simulink model "Simple_3_Model"  (R2022b)
settings: Solver=FixedStepAuto  StartTime=0.0  StopTime=1000  FixedStep=.05  RelTol=1e-3
undefined symbols (not defined in the file or in its folder): importedData
libraries: matrix_library x9
(part 1 of 2)
settings Model: SimulationMode=accelerator  Creator=hollis  LastModifiedBy=hollis
settings ModelReferenceCC: EnableRefExpFcnMdlSchedulingChecks=on

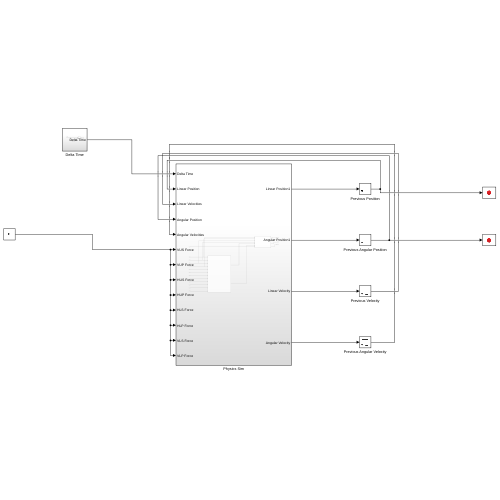
[thumbnail: Simulink's stored preview of the top-level diagram]
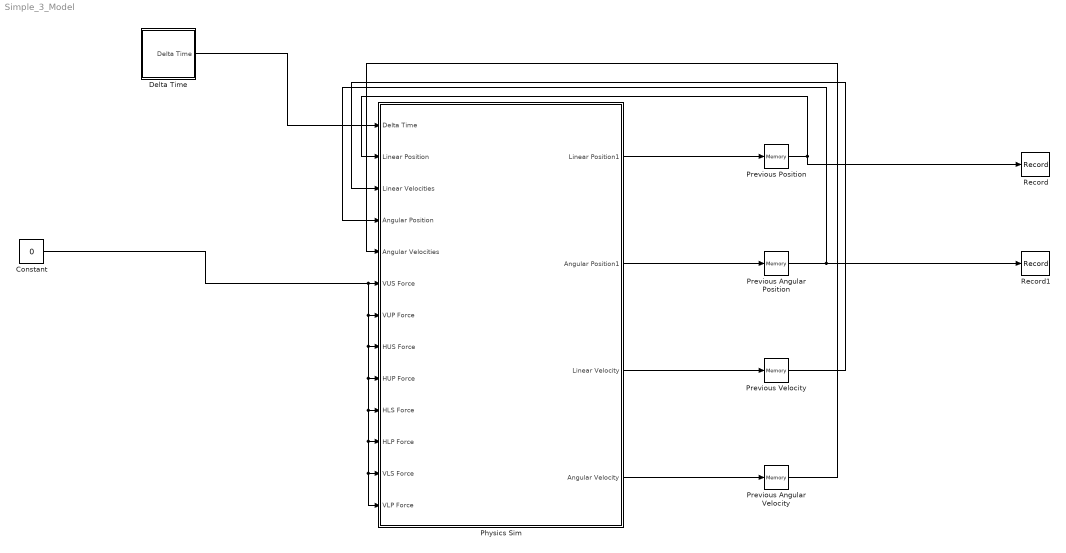
== system Simple_3_Model ==
  Constant : Constant  Value=0
  Delta Time : Subsystem
  Physics Sim : Subsystem
  Previous Angular Position : Memory
  Previous Angular Velocity : Memory
  Previous Position : Memory  InitialCondition=[0,0,-1]
  Previous Velocity : Memory
  Record : Record  FileSettingsInternal="{\"entries\":[{\"content\":{\"excelSettings\":{\"content\":{},\"type\":\"Streamout.ExcelSettings\"}},\"type\":\"Streamout.FileSettingStorage\",\"uuid\":\"11bcd66e-7632-4a96-a488-3543fce7ee1d\"}],\"packageUris\":[\"http://schema.mathworks.com/mf0/streamout_blocks/R2020a\"],\"version\":\"1.0\"}"  SignalsInternal="{\"entries\":[{\"content\":{\"signals\":[{\"content\":{\"blockPath\":[\"Simple_3_Model/Record\"],\"channel\":[],\"dimensions\":[1,3],\"domain\":\"Simple_3_Model/Record\",\"hasChildren\":true,\"lineColor\":\"#fe330a\",\"plots\":[],\"port\":1,\"sid\":[\"\"],\"signalID\":926,\"signalName\":\"Previous Position\"},\"type\":\"RecordBlkView.Signal\",\"uuid\":\"373110d8-16e4-4d5b-b50e-cea3cb7c1b6c\"},{\"content\":{\"blockPath\":[\"Simple_3_Model/Record\"],\"channel\":[1,1],\"dimensions\":[1,3],\"domain\":\"Simple_3_Model/Record\",\"lineColor\":\"#d95319\",\"parentID\":926,\"plots\":[1],\"port\":1,\"sid\":[\"\"],\"signalID\":927,\"signalName\":\"Previous Position\"},\"type\":\"RecordBlkView.Signal\",\"uuid\":\"bcdab5c0-74a8-478b-9c24-691629be9185\"},{\"content\":{\"blockPath\":[\"Simple_3_Model/Record\"],\"channel\":[1,2],\"dimensions\":[1,3],\"domain\":\"Simple_3_Model/Record\",\"lineColor\":\"#22b573\",\"parentID\":926,\"plots\":[1],\"port\":1,\"sid\":[\"\"],\"signalID\":965,\"signalName\":\"Previous Position\"},\"type\":\"RecordBlkView.Signal\",\"uuid\":\"4fc746e4-520d-4283-b26c-b6a945fd0e94\"},{\"content\":{\"blockPath\":[\"Simple_3_Model/Record\"],\"channel\":[1,3],\"dimensions\":[1,3],\"domain\":\"Simple_3_Model/Record\",\"lineColor\":\"#0072bd\",\"parentID\":926,\"plots\":[1],\"port\":1,\"sid\":[\"\"],\"signalID\":966,\"signalName\":\"Previous Position\"},\"type\":\"RecordBlkView.Signal\",\"uuid\":\"20b07a7b-441e-4fa1-b232-437ed8d86cd2\"}]},\"type\":\"RecordBlkView.InputSignals\",\"uuid\":\"0cc5a42f-1473-481d-9a59-2aee6edbe01c\"}],\"packageUris\":[\"http://schema.mathworks.com/mf0/streamout_blocks/R2020a\"],\"version\":\"1.0\"}"  VisualizationBindings="{\"sparklinesplugin\":{\"info\":[{\"bindingParametersList\":[],\"subplotID\":1}]}}"
  Record1 : Record  FileSettingsInternal="{\"entries\":[{\"content\":{\"excelSettings\":{\"content\":{},\"type\":\"Streamout.ExcelSettings\"}},\"type\":\"Streamout.FileSettingStorage\",\"uuid\":\"971a0b71-2232-4346-b6ce-2804bd4b2a6a\"}],\"packageUris\":[\"http://schema.mathworks.com/mf0/streamout_blocks/R2020a\"],\"version\":\"1.0\"}"  SignalsInternal="{\"entries\":[{\"content\":{\"signals\":[{\"content\":{\"blockPath\":[\"Simple_3_Model/Record1\"],\"channel\":[],\"dimensions\":[1,3],\"domain\":\"Simple_3_Model/Record1\",\"hasChildren\":true,\"lineColor\":\"#0072bd\",\"plots\":[],\"port\":1,\"sid\":[\"\"],\"signalID\":931,\"signalName\":\"Previous Angular Position\"},\"type\":\"RecordBlkView.Signal\",\"uuid\":\"942ad879-51dd-44a6-9b93-fffe35835e0f\"},{\"content\":{\"blockPath\":[\"Simple_3_Model/Record1\"],\"channel\":[1,1],\"dimensions\":[1,3],\"domain\":\"Simple_3_Model/Record1\",\"lineColor\":\"#0072bd\",\"parentID\":931,\"plots\":[1],\"port\":1,\"sid\":[\"\"],\"signalID\":932,\"signalName\":\"Previous Angular Position\"},\"type\":\"RecordBlkView.Signal\",\"uuid\":\"0f7508f4-6f39-4d77-9981-5362550e1fb4\"},{\"content\":{\"blockPath\":[\"Simple_3_Model/Record1\"],\"channel\":[1,2],\"dimensions\":[1,3],\"domain\":\"Simple_3_Model/Record1\",\"lineColor\":\"#0072bd\",\"parentID\":931,\"plots\":[1],\"port\":1,\"sid\":[\"\"],\"signalID\":967,\"signalName\":\"Previous Angular Position\"},\"type\":\"RecordBlkView.Signal\",\"uuid\":\"f8e5f5da-daa1-4c33-b5ed-8b7ecbecee5a\"},{\"content\":{\"blockPath\":[\"Simple_3_Model/Record1\"],\"channel\":[1,3],\"dimensions\":[1,3],\"domain\":\"Simple_3_Model/Record1\",\"lineColor\":\"#d95319\",\"parentID\":931,\"plots\":[1],\"port\":1,\"sid\":[\"\"],\"signalID\":968,\"signalName\":\"Previous Angular Position\"},\"type\":\"RecordBlkView.Signal\",\"uuid\":\"b5832108-d461-432d-a375-5bfff83e6820\"}]},\"type\":\"RecordBlkView.InputSignals\",\"uuid\":\"14037c08-81e6-44a9-86f7-5d7daad76c4f\"}],\"packageUris\":[\"http://schema.mathworks.com/mf0/streamout_blocks/R2020a\"],\"version\":\"1.0\"}"  VisualizationBindings="{\"sparklinesplugin\":{\"info\":[{\"bindingParametersList\":[],\"subplotID\":1}]}}"
  wires:
  Physics Sim/1(Linear Position1) -> Previous Position/1
  Physics Sim/2(Angular Position1) -> Previous Angular Position/1
  Physics Sim/3(Linear Velocity) -> Previous Velocity/1
  Physics Sim/4(Angular Velocity) -> Previous Angular Velocity/1
  Delta Time/1(Delta Time) -> Physics Sim/1(Delta Time)
  Previous Position/1 -> Record/1, Physics Sim/2(Linear Position)
  Previous Angular Position/1 -> Record1/1, Physics Sim/4(Angular Position)
  Previous Velocity/1 -> Physics Sim/3(Linear Velocities)
  Previous Angular Velocity/1 -> Physics Sim/5(Angular Velocities)
  Constant/1 -> Physics Sim/13(VLP Force), Physics Sim/12(VLS Force), Physics Sim/11(HLP Force), Physics Sim/10(HLS Force), Physics Sim/9(HUP Force), Physics Sim/8(HUS Force), Physics Sim/7(VUP Force), Physics Sim/6(VUS Force)

== system Simple_3_Model/Delta Time ==
  Absolute Time : Clock
  Previous Absolute : Memory
  Subtract : Sum  Inputs=+-
  Delta Time : Outport
  wires:
  Previous Absolute/1 -> Subtract/2
  Absolute Time/1 -> Subtract/1, Previous Absolute/1
  Subtract/1 -> Delta Time/1

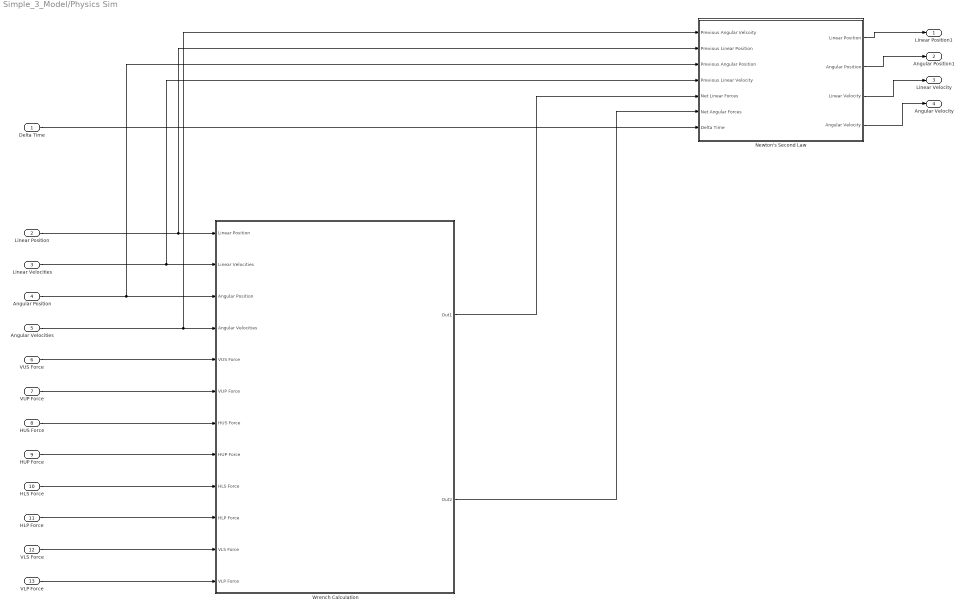
== system Simple_3_Model/Physics Sim ==
  Delta Time : Inport
  Linear Position : Inport  Port=2
  Linear Velocities : Inport  Port=3
  Angular Position : Inport  Port=4
  Angular Velocities : Inport  Port=5
  VUS Force : Inport  Port=6
  VUP Force : Inport  Port=7
  HUS Force : Inport  Port=8
  HUP Force : Inport  Port=9
  HLS Force : Inport  Port=10
  HLP Force : Inport  Port=11
  VLS Force : Inport  Port=12
  VLP Force : Inport  Port=13
  Newton's Second Law : Subsystem
  Wrench Calculation : Subsystem
  Linear Position1 : Outport
  Angular Position1 : Outport  Port=2
  Linear Velocity : Outport  Port=3
  Angular Velocity : Outport  Port=4
  wires:
  Delta Time/1 -> Newton's Second Law/7(Delta Time)
  VLP Force/1 -> Wrench Calculation/12(VLP Force)
  VUP Force/1 -> Wrench Calculation/6(VUP Force)
  Newton's Second Law/3(Linear Velocity) -> Linear Velocity/1
  VUS Force/1 -> Wrench Calculation/5(VUS Force)
  Newton's Second Law/1(Linear Position) -> Linear Position1/1
  Newton's Second Law/4(Angular Velocity) -> Angular Velocity/1
  HLS Force/1 -> Wrench Calculation/9(HLS Force)
  Angular Position/1 -> Newton's Second Law/3(Previous Angular Position), Wrench Calculation/3(Angular Position)
  Newton's Second Law/2(Angular Position) -> Angular Position1/1
  VLS Force/1 -> Wrench Calculation/11(VLS Force)
  HLP Force/1 -> Wrench Calculation/10(HLP Force)
  HUP Force/1 -> Wrench Calculation/8(HUP Force)
  Angular Velocities/1 -> Newton's Second Law/1(Previous Angular Velcoity), Wrench Calculation/4(Angular Velocities)
  Linear Velocities/1 -> Newton's Second Law/4(Previous Linear Velocity), Wrench Calculation/2(Linear Velocities)
  Wrench Calculation/1(Out1) -> Newton's Second Law/5(Net Linear Forces)
  Linear Position/1 -> Newton's Second Law/2(Previous Linear Position), Wrench Calculation/1(Linear Position)
  HUS Force/1 -> Wrench Calculation/7(HUS Force)
  Wrench Calculation/2(Out2) -> Newton's Second Law/6(Net Angular Forces)

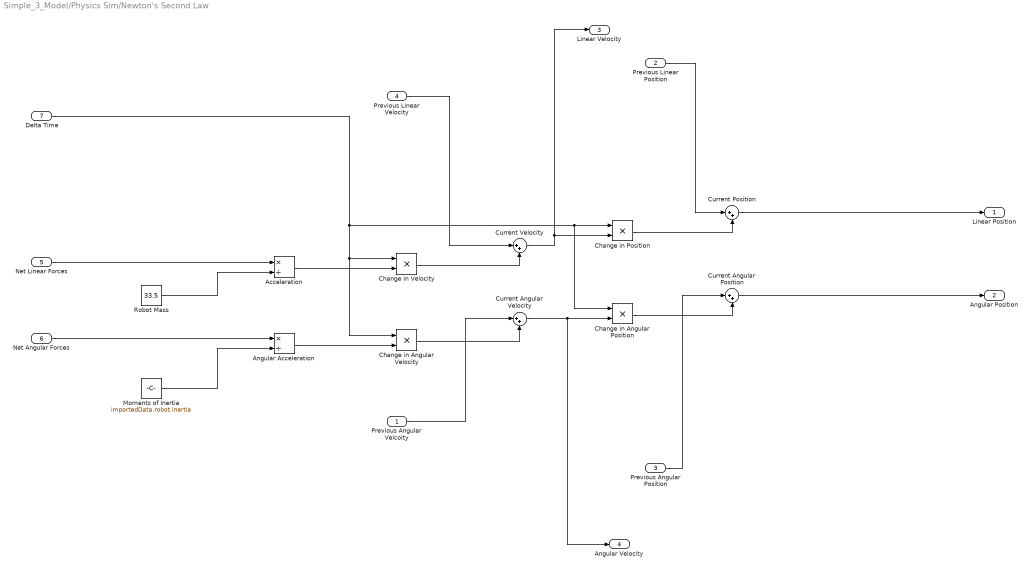
== system Simple_3_Model/Physics Sim/Newton's Second Law ==
  Previous Angular Velcoity : Inport
  Previous Linear Position : Inport  Port=2
  Previous Angular Position : Inport  Port=3
  Previous Linear Velocity : Inport  Port=4
  Net Linear Forces : Inport  Port=5
  Net Angular Forces : Inport  Port=6
  Delta Time : Inport  Port=7
  Acceleration : Product  Inputs=*/
  Angular Acceleration : Product  Inputs=*/
  Change in Angular Position : Product
  Change in Angular Velocity : Product
  Change in Position : Product
  Change in Velocity : Product
  Current Angular Position : Sum  Inputs=|++
  Current Angular Velocity : Sum  Inputs=|++
  Current Position : Sum  Inputs=|++
  Current Velocity : Sum  Inputs=|++
  Moments of Inertia : Constant  Value=importedData.robot.inertia  VectorParams1D=off
  Robot Mass : Constant  Value=33.5
  Linear Position : Outport
  Angular Position : Outport  Port=2
  Linear Velocity : Outport  Port=3
  Angular Velocity : Outport  Port=4
  wires:
  Current Angular Position/1 -> Angular Position/1
  Acceleration/1 -> Change in Velocity/2
  Angular Acceleration/1 -> Change in Angular Velocity/2
  Change in Position/1 -> Current Position/2
  Moments of Inertia/1 -> Angular Acceleration/2
  Current Velocity/1 -> Linear Velocity/1, Change in Position/2
  Current Position/1 -> Linear Position/1
  Previous Linear Velocity/1 -> Current Velocity/1
  Change in Angular Velocity/1 -> Current Angular Velocity/2
  Net Linear Forces/1 -> Acceleration/1
  Net Angular Forces/1 -> Angular Acceleration/1
  Current Angular Velocity/1 -> Angular Velocity/1, Change in Angular Position/2
  Change in Angular Position/1 -> Current Angular Position/2
  Previous Angular Velcoity/1 -> Current Angular Velocity/1
  Delta Time/1 -> Change in Angular Velocity/1, Change in Velocity/1, Change in Angular Position/1, Change in Position/1
  Previous Linear Position/1 -> Current Position/1
  Robot Mass/1 -> Acceleration/2
  Previous Angular Position/1 -> Current Angular Position/1
  Change in Velocity/1 -> Current Velocity/2

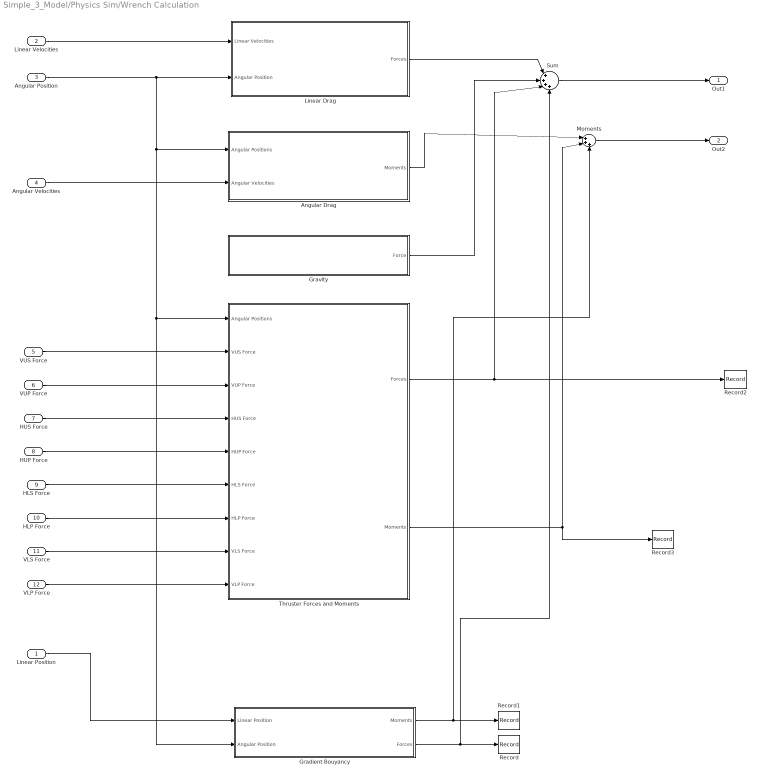
== system Simple_3_Model/Physics Sim/Wrench Calculation ==
  Linear Position : Inport
  Linear Velocities : Inport  Port=2
  Angular Position : Inport  Port=3
  Angular Velocities : Inport  Port=4
  VUS Force : Inport  Port=5
  VUP Force : Inport  Port=6
  HUS Force : Inport  Port=7
  HUP Force : Inport  Port=8
  HLS Force : Inport  Port=9
  HLP Force : Inport  Port=10
  VLS Force : Inport  Port=11
  VLP Force : Inport  Port=12
  Angular Drag : Subsystem
  Gradient Bouyancy : Subsystem
  Gravity : Subsystem
  Linear Drag : Subsystem
  Moments : Sum  Inputs=|+++
  Record : Record  FileSettingsInternal="{\"entries\":[{\"content\":{\"excelSettings\":{\"content\":{},\"type\":\"Streamout.ExcelSettings\"}},\"type\":\"Streamout.FileSettingStorage\",\"uuid\":\"14ae8275-bff0-4191-85a7-8bdbe692570f\"}],\"packageUris\":[\"http://schema.mathworks.com/mf0/streamout_blocks/R2020a\"],\"version\":\"1.0\"}"  SignalsInternal="{\"entries\":[{\"content\":{\"signals\":[{\"content\":{\"blockPath\":[\"Simple_3_Model/Physics Sim/Wrench Calculation/Record\"],\"channel\":[],\"dimensions\":[1,3],\"domain\":\"Simple_3_Model/Physics Sim/Wrench Calculation/Record\",\"hasChildren\":true,\"lineColor\":\"#edb120\",\"plots\":[],\"port\":1,\"sid\":[\"\"],\"signalID\":936,\"signalName\":\"Gradient Bouyancy:2\"},\"type\":\"RecordBlkView.Signal\",\"uuid\":\"7bfce770-828e-487e-b922-719935c79236\"},{\"content\":{\"blockPath\":[\"Simple_3_Model/Physics Sim/Wrench Calculation/Record\"],\"channel\":[1,1],\"dimensions\":[1,3],\"domain\":\"Simple_3_Model/Physics Sim/Wrench Calculation/Record\",\"lineColor\":\"#ff6929\",\"parentID\":936,\"plots\":[1],\"port\":1,\"sid\":[\"\"],\"signalID\":937,\"signalName\":\"Gradient Bouyancy:2\"},\"type\":\"RecordBlkView.Signal\",\"uuid\":\"0b18444a-b670-4689-ba02-5d1e4877daca\"},{\"content\":{\"blockPath\":[\"Simple_3_Model/Physics Sim/Wrench Calculation/Record\"],\"channel\":[1,2],\"dimensions\":[1,3],\"domain\":\"Simple_3_Model/Physics Sim/Wrench Calculation/Record\",\"lineColor\":\"#4dbeee\",\"parentID\":936,\"plots\":[1],\"port\":1,\"sid\":[\"\"],\"signalID\":969,\"signalName\":\"Gradient Bouyancy:2\"},\"type\":\"RecordBlkView.Signal\",\"uuid\":\"a577dcb4-3a6d-43f4-9b39-8c81b2194628\"},{\"content\":{\"blockPath\":[\"Simple_3_Model/Physics Sim/Wrench Calculation/Record\"],\"channel\":[1,3],\"dimensions\":[1,3],\"domain\":\"Simple_3_Model/Physics Sim/Wrench Calculation/Record\",\"lineColor\":\"#a2142f\",\"parentID\":936,\"plots\":[1],\"port\":1,\"sid\":[\"\"],\"signalID\":970,\"signalName\":\"Gradient Bouyancy:2\"},\"type\":\"RecordBlkView.Signal\",\"uuid\":\"bcba812b-f663-473e-a7f6-fe747fcb18b0\"}]},\"type\":\"RecordBlkView.InputSignals\",\"uuid\":\"80eec240-2a13-4c7e-96b9-5123065623d5\"}],\"packageUris\":[\"http://schema.mathworks.com/mf0/streamout_blocks/R2020a\"],\"version\":\"1.0\"}"  VisualizationBindings="{\"sparklinesplugin\":{\"info\":[{\"bindingParametersList\":[],\"subplotID\":1}]}}"
  Record1 : Record  FileSettingsInternal="{\"entries\":[{\"content\":{\"excelSettings\":{\"content\":{},\"type\":\"Streamout.ExcelSettings\"}},\"type\":\"Streamout.FileSettingStorage\",\"uuid\":\"c8ebd48f-3dda-4790-90f8-fdd6d3865a6d\"}],\"packageUris\":[\"http://schema.mathworks.com/mf0/streamout_blocks/R2020a\"],\"version\":\"1.0\"}"  SignalsInternal="{\"entries\":[{\"content\":{\"signals\":[{\"content\":{\"blockPath\":[\"Simple_3_Model/Physics Sim/Wrench Calculation/Record1\"],\"channel\":[],\"dimensions\":[1,3],\"domain\":\"Simple_3_Model/Physics Sim/Wrench Calculation/Record1\",\"hasChildren\":true,\"lineColor\":\"#77ac30\",\"plots\":[],\"port\":1,\"sid\":[\"\"],\"signalID\":941,\"signalName\":\"Gradient Bouyancy:1\"},\"type\":\"RecordBlkView.Signal\",\"uuid\":\"01770711-47fc-4378-9b06-d566efdae185\"},{\"content\":{\"blockPath\":[\"Simple_3_Model/Physics Sim/Wrench Calculation/Record1\"],\"channel\":[1,1],\"dimensions\":[1,3],\"domain\":\"Simple_3_Model/Physics Sim/Wrench Calculation/Record1\",\"lineColor\":\"#64d413\",\"parentID\":941,\"plots\":[1],\"port\":1,\"sid\":[\"\"],\"signalID\":942,\"signalName\":\"Gradient Bouyancy:1\"},\"type\":\"RecordBlkView.Signal\",\"uuid\":\"9acf9cb1-4fa8-4bf8-90f0-6f697aa656da\"},{\"content\":{\"blockPath\":[\"Simple_3_Model/Physics Sim/Wrench Calculation/Record1\"],\"channel\":[1,2],\"dimensions\":[1,3],\"domain\":\"Simple_3_Model/Physics Sim/Wrench Calculation/Record1\",\"lineColor\":\"#139fff\",\"parentID\":941,\"plots\":[1],\"port\":1,\"sid\":[\"\"],\"signalID\":971,\"signalName\":\"Gradient Bouyancy:1\"},\"type\":\"RecordBlkView.Signal\",\"uuid\":\"442f376c-a923-410e-a81f-817bbf379f20\"},{\"content\":{\"blockPath\":[\"Simple_3_Model/Physics Sim/Wrench Calculation/Record1\"],\"channel\":[1,3],\"dimensions\":[1,3],\"domain\":\"Simple_3_Model/Physics Sim/Wrench Calculation/Record1\",\"lineColor\":\"#ff6929\",\"parentID\":941,\"plots\":[1],\"port\":1,\"sid\":[\"\"],\"signalID\":972,\"signalName\":\"Gradient Bouyancy:1\"},\"type\":\"RecordBlkView.Signal\",\"uuid\":\"d23a1b4a-4761-4174-b835-0283a7d905c5\"}]},\"type\":\"RecordBlkView.InputSignals\",\"uuid\":\"540da4e7-907c-4693-a7c6-038eda139879\"}],\"packageUris\":[\"http://schema.mathworks.com/mf0/streamout_blocks/R2020a\"],\"version\":\"1.0\"}"  VisualizationBindings="{\"sparklinesplugin\":{\"info\":[{\"bindingParametersList\":[],\"subplotID\":1}]}}"
  Record2 : Record  FileSettingsInternal="{\"entries\":[{\"content\":{\"excelSettings\":{\"content\":{},\"type\":\"Streamout.ExcelSettings\"}},\"type\":\"Streamout.FileSettingStorage\",\"uuid\":\"6320329a-b3d7-4a3d-9256-9fc55a292c12\"}],\"packageUris\":[\"http://schema.mathworks.com/mf0/streamout_blocks/R2020a\"],\"version\":\"1.0\"}"  SignalsInternal="{\"entries\":[{\"content\":{\"signals\":[{\"content\":{\"blockPath\":[\"Simple_3_Model/Physics Sim/Wrench Calculation/Record2\"],\"channel\":[],\"dimensions\":[1,3],\"domain\":\"Simple_3_Model/Physics Sim/Wrench Calculation/Record2\",\"hasChildren\":true,\"lineColor\":\"#a2142f\",\"plots\":[],\"port\":1,\"sid\":[\"\"],\"signalID\":946,\"signalName\":\"Thruster Forces and Moments:1\"},\"type\":\"RecordBlkView.Signal\",\"uuid\":\"e0bec64a-e0fc-4c30-ba04-1f75709ad5d1\"},{\"content\":{\"blockPath\":[\"Simple_3_Model/Physics Sim/Wrench Calculation/Record2\"],\"channel\":[1,1],\"dimensions\":[1,3],\"domain\":\"Simple_3_Model/Physics Sim/Wrench Calculation/Record2\",\"lineColor\":\"#0072bd\",\"parentID\":946,\"plots\":[1],\"port\":1,\"sid\":[\"\"],\"signalID\":947,\"signalName\":\"Thruster Forces and Moments:1\"},\"type\":\"RecordBlkView.Signal\",\"uuid\":\"92f7a7a3-98ca-4f61-a9f6-ac5a2e273ed5\"},{\"content\":{\"blockPath\":[\"Simple_3_Model/Physics Sim/Wrench Calculation/Record2\"],\"channel\":[1,2],\"dimensions\":[1,3],\"domain\":\"Simple_3_Model/Physics Sim/Wrench Calculation/Record2\",\"lineColor\":\"#ff6929\",\"parentID\":946,\"plots\":[1],\"port\":1,\"sid\":[\"\"],\"signalID\":973,\"signalName\":\"Thruster Forces and Moments:1\"},\"type\":\"RecordBlkView.Signal\",\"uuid\":\"18811a90-2073-45f0-bfd8-044204d09150\"},{\"content\":{\"blockPath\":[\"Simple_3_Model/Physics Sim/Wrench Calculation/Record2\"],\"channel\":[1,3],\"dimensions\":[1,3],\"domain\":\"Simple_3_Model/Physics Sim/Wrench Calculation/Record2\",\"lineColor\":\"#b746ff\",\"parentID\":946,\"plots\":[1],\"port\":1,\"sid\":[\"\"],\"signalID\":974,\"signalName\":\"Thruster Forces and Moments:1\"},\"type\":\"RecordBlkView.Signal\",\"uuid\":\"9b6661de-aa9e-465a-9956-bf3c252ad696\"}]},\"type\":\"RecordBlkView.InputSignals\",\"uuid\":\"99ab9542-22fb-43c8-8711-76634d927cda\"}],\"packageUris\":[\"http://schema.mathworks.com/mf0/streamout_blocks/R2020a\"],\"version\":\"1.0\"}"  VisualizationBindings="{\"sparklinesplugin\":{\"info\":[{\"bindingParametersList\":[],\"subplotID\":1}]}}"
  Record3 : Record  FileSettingsInternal="{\"entries\":[{\"content\":{\"excelSettings\":{\"content\":{},\"type\":\"Streamout.ExcelSettings\"}},\"type\":\"Streamout.FileSettingStorage\",\"uuid\":\"735e6848-6a90-4887-87fc-d3808a9da643\"}],\"packageUris\":[\"http://schema.mathworks.com/mf0/streamout_blocks/R2020a\"],\"version\":\"1.0\"}"  SignalsInternal="{\"entries\":[{\"content\":{\"signals\":[{\"content\":{\"blockPath\":[\"Simple_3_Model/Physics Sim/Wrench Calculation/Record3\"],\"channel\":[],\"dimensions\":[1,3],\"domain\":\"Simple_3_Model/Physics Sim/Wrench Calculation/Record3\",\"hasChildren\":true,\"lineColor\":\"#ff6929\",\"plots\":[],\"port\":1,\"sid\":[\"\"],\"signalID\":951,\"signalName\":\"Thruster Forces and Moments:2\"},\"type\":\"RecordBlkView.Signal\",\"uuid\":\"2fec76c9-c181-44a4-8562-f7d80885c062\"},{\"content\":{\"blockPath\":[\"Simple_3_Model/Physics Sim/Wrench Calculation/Record3\"],\"channel\":[1,1],\"dimensions\":[1,3],\"domain\":\"Simple_3_Model/Physics Sim/Wrench Calculation/Record3\",\"lineColor\":\"#fe330a\",\"parentID\":951,\"plots\":[1],\"port\":1,\"sid\":[\"\"],\"signalID\":952,\"signalName\":\"Thruster Forces and Moments:2\"},\"type\":\"RecordBlkView.Signal\",\"uuid\":\"24551375-e6ba-49cc-8583-5af06021d20b\"},{\"content\":{\"blockPath\":[\"Simple_3_Model/Physics Sim/Wrench Calculation/Record3\"],\"channel\":[1,2],\"dimensions\":[1,3],\"domain\":\"Simple_3_Model/Physics Sim/Wrench Calculation/Record3\",\"lineColor\":\"#fe330a\",\"parentID\":951,\"plots\":[1],\"port\":1,\"sid\":[\"\"],\"signalID\":975,\"signalName\":\"Thruster Forces and Moments:2\"},\"type\":\"RecordBlkView.Signal\",\"uuid\":\"24a729dc-d8b1-420d-a747-ad3adf661dd4\"},{\"content\":{\"blockPath\":[\"Simple_3_Model/Physics Sim/Wrench Calculation/Record3\"],\"channel\":[1,3],\"dimensions\":[1,3],\"domain\":\"Simple_3_Model/Physics Sim/Wrench Calculation/Record3\",\"lineColor\":\"#22b573\",\"parentID\":951,\"plots\":[1],\"port\":1,\"sid\":[\"\"],\"signalID\":976,\"signalName\":\"Thruster Forces and Moments:2\"},\"type\":\"RecordBlkView.Signal\",\"uuid\":\"db5cf133-f132-4155-8865-db0c13c21034\"}]},\"type\":\"RecordBlkView.InputSignals\",\"uuid\":\"ca0fbc76-8d67-43df-b7b5-547daaad5820\"}],\"packageUris\":[\"http://schema.mathworks.com/mf0/streamout_blocks/R2020a\"],\"version\":\"1.0\"}"  VisualizationBindings="{\"sparklinesplugin\":{\"info\":[{\"bindingParametersList\":[],\"subplotID\":1}]}}"
  Sum : Sum  Inputs=|++++
  Thruster Forces and Moments : Subsystem
  Out1 : Outport
  Out2 : Outport  Port=2
  wires:
  Thruster Forces and Moments/1(Forces) -> Record2/1, Sum/3
  Angular Drag/1(Moments) -> Moments/1
  Thruster Forces and Moments/2(Moments) -> Moments/2, Record3/1
  Gradient Bouyancy/2(Forces) -> Sum/4, Record/1
  Gradient Bouyancy/1(Moments) -> Moments/3, Record1/1
  HLP Force/1 -> Thruster Forces and Moments/7(HLP Force)
  Sum/1 -> Out1/1
  Angular Position/1 -> Linear Drag/2(Angular Position), Angular Drag/1(Angular Positions), Gradient Bouyancy/2(Angular Position), Thruster Forces and Moments/1(Angular Positions)
  Linear Position/1 -> Gradient Bouyancy/1(Linear Position)
  Linear Drag/1(Forces) -> Sum/1
  HUP Force/1 -> Thruster Forces and Moments/5(HUP Force)
  VLP Force/1 -> Thruster Forces and Moments/9(VLP Force)
  VUS Force/1 -> Thruster Forces and Moments/2(VUS Force)
  VUP Force/1 -> Thruster Forces and Moments/3(VUP Force)
  Gravity/1(Force) -> Sum/2
  VLS Force/1 -> Thruster Forces and Moments/8(VLS Force)
  Moments/1 -> Out2/1
  HLS Force/1 -> Thruster Forces and Moments/6(HLS Force)
  Linear Velocities/1 -> Linear Drag/1(Linear Velocities)
  HUS Force/1 -> Thruster Forces and Moments/4(HUS Force)
  Angular Velocities/1 -> Angular Drag/2(Angular Velocities)

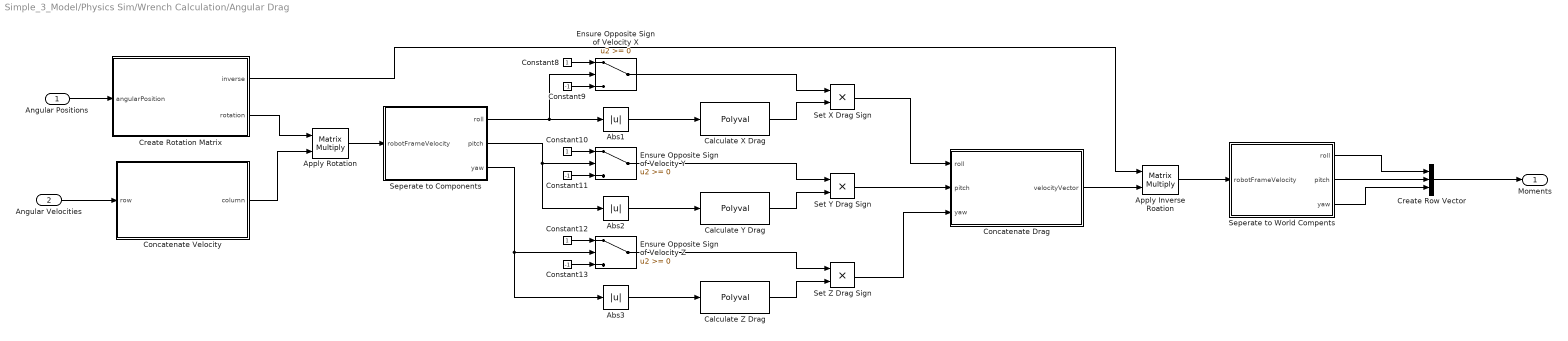
== system Simple_3_Model/Physics Sim/Wrench Calculation/Angular Drag ==
  Angular Positions : Inport
  Angular Velocities : Inport  Port=2
  Abs1 : Abs  SaturateOnIntegerOverflow=off
  Abs2 : Abs  SaturateOnIntegerOverflow=off
  Abs3 : Abs  SaturateOnIntegerOverflow=off
  Apply Inverse Roation : Product  Multiplication=Matrix(*)
  Apply Rotation : Product  Multiplication=Matrix(*)
  Calculate X Drag : Polyval  Coefs=importedData.robot.coefficients.roll
  Calculate Y Drag : Polyval  Coefs=importedData.robot.coefficients.pitch
  Calculate Z Drag : Polyval  Coefs=importedData.robot.coefficients.yaw
  Concatenate Drag : MATLAB Function  TreatAsAtomicUnit=on
  Concatenate Velocity : MATLAB Function  TreatAsAtomicUnit=on
  Constant10 : Constant
  Constant11 : Constant  Value=-1
  Constant12 : Constant
  Constant13 : Constant  Value=-1
  Constant8 : Constant
  Constant9 : Constant  Value=-1
  Create Rotation Matrix : MATLAB Function  TreatAsAtomicUnit=on
  Create Row Vector : Mux  Inputs=3
  Ensure Opposite Sign of Velocity X : Switch  SaturateOnIntegerOverflow=off  InputSameDT=off
  Ensure Opposite Sign of Velocity Y : Switch  SaturateOnIntegerOverflow=off  InputSameDT=off
  Ensure Opposite Sign of Velocity Z : Switch  SaturateOnIntegerOverflow=off  InputSameDT=off
  Seperate to Components : MATLAB Function  TreatAsAtomicUnit=on
  Seperate to World Compents : MATLAB Function  TreatAsAtomicUnit=on
  Set X Drag Sign : Product
  Set Y Drag Sign : Product
  Set Z Drag Sign : Product
  Moments : Outport
  wires:
  Concatenate Drag/1(velocityVector) -> Apply Inverse Roation/2
  Calculate Y Drag/1 -> Set Y Drag Sign/2
  Constant11/1 -> Ensure Opposite Sign of Velocity Y/3
  Calculate Z Drag/1 -> Set Z Drag Sign/2
  Abs1/1 -> Calculate X Drag/1
  Apply Rotation/1 -> Seperate to Components/1(robotFrameVelocity)
  Apply Inverse Roation/1 -> Seperate to World Compents/1(robotFrameVelocity)
  Angular Velocities/1 -> Concatenate Velocity/1(row)
  Constant8/1 -> Ensure Opposite Sign of Velocity X/1
  Set Z Drag Sign/1 -> Concatenate Drag/3(yaw)
  Constant13/1 -> Ensure Opposite Sign of Velocity Z/3
  Constant9/1 -> Ensure Opposite Sign of Velocity X/3
  Set Y Drag Sign/1 -> Concatenate Drag/2(pitch)
  Ensure Opposite Sign of Velocity Y/1 -> Set Y Drag Sign/1
  Seperate to Components/2(pitch) -> Abs2/1, Ensure Opposite Sign of Velocity Y/2
  Set X Drag Sign/1 -> Concatenate Drag/1(roll)
  Seperate to World Compents/3(yaw) -> Create Row Vector/3
  Constant12/1 -> Ensure Opposite Sign of Velocity Z/1
  Create Rotation Matrix/2(rotation) -> Apply Rotation/1
  Concatenate Velocity/1(column) -> Apply Rotation/2
  Seperate to World Compents/1(roll) -> Create Row Vector/1
  Ensure Opposite Sign of Velocity X/1 -> Set X Drag Sign/1
  Seperate to Components/1(roll) -> Ensure Opposite Sign of Velocity X/2, Abs1/1
  Seperate to World Compents/2(pitch) -> Create Row Vector/2
  Create Rotation Matrix/1(inverse) -> Apply Inverse Roation/1
  Constant10/1 -> Ensure Opposite Sign of Velocity Y/1
  Calculate X Drag/1 -> Set X Drag Sign/2
  Abs2/1 -> Calculate Y Drag/1
  Abs3/1 -> Calculate Z Drag/1
  Seperate to Components/3(yaw) -> Ensure Opposite Sign of Velocity Z/2, Abs3/1
  Ensure Opposite Sign of Velocity Z/1 -> Set Z Drag Sign/1
  Create Row Vector/1 -> Moments/1
  Angular Positions/1 -> Create Rotation Matrix/1(angularPosition)

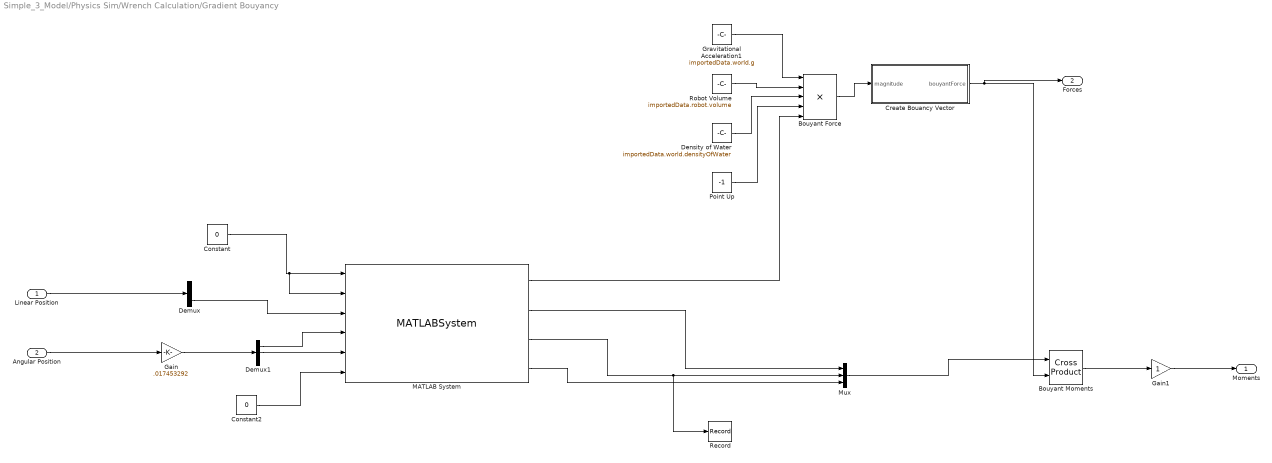
== system Simple_3_Model/Physics Sim/Wrench Calculation/Gradient Bouyancy ==
  Linear Position : Inport
  Angular Position : Inport  Port=2
  Bouyant Force : Product  Inputs=5
  Bouyant Moments : matrix_library/Cross Product
  Constant : Constant  Value=0
  Constant2 : Constant  Value=0
  Create Bouancy Vector : MATLAB Function  TreatAsAtomicUnit=on
  Demux : Demux  Outputs=3
  Demux1 : Demux  Outputs=3
  Density of Water : Constant  Value=importedData.world.densityOfWater
  Gain : Gain  Gain=.017453292
  Gain1 : Gain
  Gravitational Acceleration1 : Constant  Value=importedData.world.g
  MATLAB System : MATLABSystem  System=GradientBouyancySystem  SimulateUsing=Interpreted execution
      mask Type: GradientBouyancySystem
      mask Display:
      | disp('GradientBouyancySystem');
      | port_label('input',1,'x_position');
      | port_label('input',2,'y_position');
      | port_label('input',3,'z_position');
      | port_label('input',4,'roll');
      | port_label('input',5,'pitch');
      | port_label('input',6,'yaw');
      | port_label('output',1,'force');
      | port_label('output',2,'x_acting');
      | port_label('output',3,'y_acting');
      | port_label('output',4,'z_acting');
  Mux : Mux  Inputs=3
  Point Up : Constant  Value=-1
  Record : Record  FileSettingsInternal="{\"entries\":[{\"content\":{\"excelSettings\":{\"content\":{},\"type\":\"Streamout.ExcelSettings\"}},\"type\":\"Streamout.FileSettingStorage\",\"uuid\":\"43d747a8-ad29-43c8-a0d8-60c09ebb7318\"}],\"packageUris\":[\"http://schema.mathworks.com/mf0/streamout_blocks/R2020a\"],\"version\":\"1.0\"}"  SignalsInternal="{\"entries\":[{\"content\":{\"signals\":[{\"content\":{\"blockPath\":[\"Simple_3_Model/Physics Sim/Wrench Calculation/Gradient Bouyancy/Record\"],\"channel\":[],\"dimensions\":[1,1],\"domain\":\"Simple_3_Model/Physics Sim/Wrench Calculation/Gradient Bouyancy/Record\",\"lineColor\":\"#7e2f8e\",\"plots\":[1],\"port\":1,\"sid\":[\"\"],\"signalID\":956,\"signalName\":\"MATLAB System:3\"},\"type\":\"RecordBlkView.Signal\",\"uuid\":\"9cbb49a7-6a7d-4414-8002-013d14d0a626\"}]},\"type\":\"RecordBlkView.InputSignals\",\"uuid\":\"7b021675-76e6-44e5-a82b-815b9bd86361\"}],\"packageUris\":[\"http://schema.mathworks.com/mf0/streamout_blocks/R2020a\"],\"version\":\"1.0\"}"  VisualizationBindings="{\"sparklinesplugin\":{\"info\":[{\"bindingParametersList\":[],\"subplotID\":1}]}}"
  Robot Volume : Constant  Value=importedData.robot.volume
  Moments : Outport
  Forces : Outport  Port=2
  wires:
  Density of Water/1 -> Bouyant Force/3
  Gravitational Acceleration1/1 -> Bouyant Force/1
  Bouyant Force/1 -> Create Bouancy Vector/1(magnitude)
  Create Bouancy Vector/1(bouyantForce) -> Bouyant Moments/2, Forces/1
  Robot Volume/1 -> Bouyant Force/2
  Bouyant Moments/1 -> Gain1/1
  Point Up/1 -> Bouyant Force/4
  MATLAB System/1 -> Bouyant Force/5
  Demux/3 -> MATLAB System/3
  Angular Position/1 -> Gain/1
  Demux1/1 -> MATLAB System/4
  Demux1/2 -> MATLAB System/5
  Mux/1 -> Bouyant Moments/1
  MATLAB System/2 -> Mux/1
  MATLAB System/3 -> Record/1, Mux/2
  Gain/1 -> Demux1/1
  Gain1/1 -> Moments/1
  Constant2/1 -> MATLAB System/6
  MATLAB System/4 -> Mux/3
  Linear Position/1 -> Demux/1
  Constant/1 -> MATLAB System/2, MATLAB System/1

== system Simple_3_Model/Physics Sim/Wrench Calculation/Gravity ==
  Create Vector : MATLAB Function  TreatAsAtomicUnit=on
  Gravitational Acceleration1 : Constant  Value=importedData.world.g
  Gravitational Force1 : Product
  Robot Mass : Constant  Value=importedData.robot.mass
  Force : Outport
  wires:
  Gravitational Acceleration1/1 -> Gravitational Force1/1
  Robot Mass/1 -> Gravitational Force1/2
  Create Vector/1(vector) -> Force/1
  Gravitational Force1/1 -> Create Vector/1(magnitude)

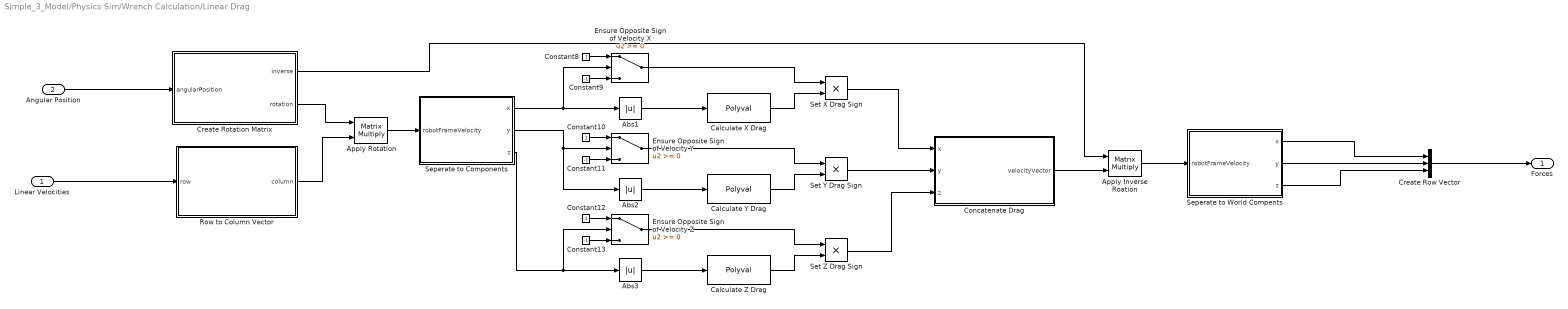
== system Simple_3_Model/Physics Sim/Wrench Calculation/Linear Drag ==
  Linear Velocities : Inport
  Angular Position : Inport  Port=2
  Abs1 : Abs  SaturateOnIntegerOverflow=off
  Abs2 : Abs  SaturateOnIntegerOverflow=off
  Abs3 : Abs  SaturateOnIntegerOverflow=off
  Apply Inverse Roation : Product  Multiplication=Matrix(*)
  Apply Rotation : Product  Multiplication=Matrix(*)
  Calculate X Drag : Polyval  Coefs=importedData.robot.coefficients.x
  Calculate Y Drag : Polyval  Coefs=importedData.robot.coefficients.y
  Calculate Z Drag : Polyval  Coefs=importedData.robot.coefficients.z
  Concatenate Drag : MATLAB Function  TreatAsAtomicUnit=on
  Constant10 : Constant
  Constant11 : Constant  Value=-1
  Constant12 : Constant
  Constant13 : Constant  Value=-1
  Constant8 : Constant
  Constant9 : Constant  Value=-1
  Create Rotation Matrix : MATLAB Function  TreatAsAtomicUnit=on
  Create Row Vector : Mux  Inputs=3
  Ensure Opposite Sign of Velocity X : Switch  SaturateOnIntegerOverflow=off  InputSameDT=off
  Ensure Opposite Sign of Velocity Y : Switch  SaturateOnIntegerOverflow=off  InputSameDT=off
  Ensure Opposite Sign of Velocity Z : Switch  SaturateOnIntegerOverflow=off  InputSameDT=off
  Row to Column Vector : MATLAB Function  TreatAsAtomicUnit=on
  Seperate to Components : MATLAB Function  TreatAsAtomicUnit=on
  Seperate to World Compents : MATLAB Function  TreatAsAtomicUnit=on
  Set X Drag Sign : Product
  Set Y Drag Sign : Product
  Set Z Drag Sign : Product
  Forces : Outport
  wires:
  Calculate X Drag/1 -> Set X Drag Sign/2
  Ensure Opposite Sign of Velocity X/1 -> Set X Drag Sign/1
  Constant12/1 -> Ensure Opposite Sign of Velocity Z/1
  Abs2/1 -> Calculate Y Drag/1
  Constant8/1 -> Ensure Opposite Sign of Velocity X/1
  Seperate to Components/3(z) -> Abs3/1, Ensure Opposite Sign of Velocity Z/2
  Set Z Drag Sign/1 -> Concatenate Drag/3(z)
  Abs3/1 -> Calculate Z Drag/1
  Abs1/1 -> Calculate X Drag/1
  Concatenate Drag/1(velocityVector) -> Apply Inverse Roation/2
  Calculate Y Drag/1 -> Set Y Drag Sign/2
  Apply Inverse Roation/1 -> Seperate to World Compents/1(robotFrameVelocity)
  Constant9/1 -> Ensure Opposite Sign of Velocity X/3
  Constant13/1 -> Ensure Opposite Sign of Velocity Z/3
  Create Rotation Matrix/1(inverse) -> Apply Inverse Roation/1
  Create Rotation Matrix/2(rotation) -> Apply Rotation/1
  Row to Column Vector/1(column) -> Apply Rotation/2
  Constant10/1 -> Ensure Opposite Sign of Velocity Y/1
  Seperate to Components/2(y) -> Abs2/1, Ensure Opposite Sign of Velocity Y/2
  Seperate to Components/1(x) -> Abs1/1, Ensure Opposite Sign of Velocity X/2
  Constant11/1 -> Ensure Opposite Sign of Velocity Y/3
  Apply Rotation/1 -> Seperate to Components/1(robotFrameVelocity)
  Calculate Z Drag/1 -> Set Z Drag Sign/2
  Angular Position/1 -> Create Rotation Matrix/1(angularPosition)
  Ensure Opposite Sign of Velocity Y/1 -> Set Y Drag Sign/1
  Set Y Drag Sign/1 -> Concatenate Drag/2(y)
  Set X Drag Sign/1 -> Concatenate Drag/1(x)
  Ensure Opposite Sign of Velocity Z/1 -> Set Z Drag Sign/1
  Seperate to World Compents/2(y) -> Create Row Vector/2
  Seperate to World Compents/1(x) -> Create Row Vector/1
  Seperate to World Compents/3(z) -> Create Row Vector/3
  Create Row Vector/1 -> Forces/1
  Linear Velocities/1 -> Row to Column Vector/1(row)

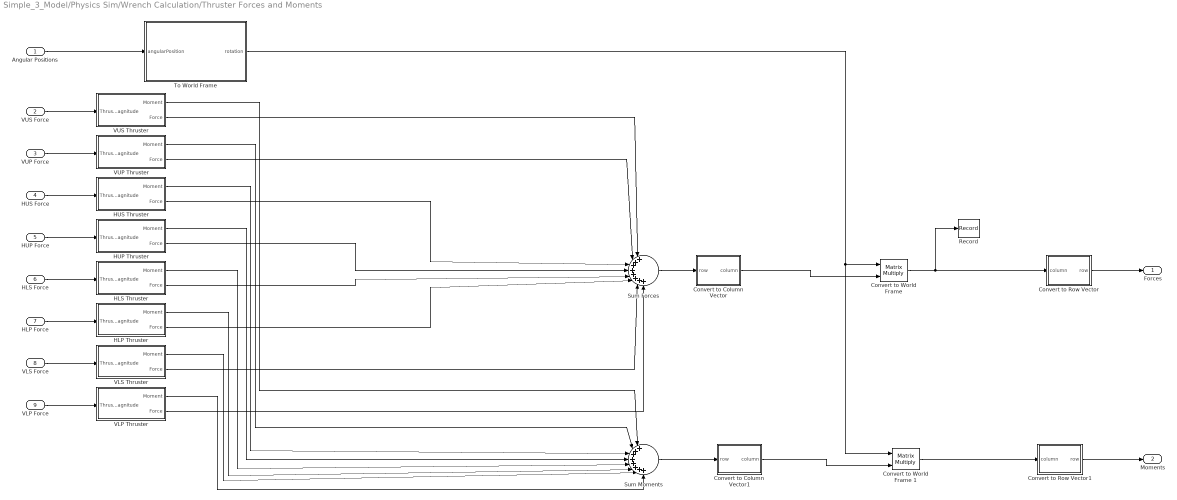
== system Simple_3_Model/Physics Sim/Wrench Calculation/Thruster Forces and Moments ==
  Angular Positions : Inport
  VUS Force : Inport  Port=2
  VUP Force : Inport  Port=3
  HUS Force : Inport  Port=4
  HUP Force : Inport  Port=5
  HLS Force : Inport  Port=6
  HLP Force : Inport  Port=7
  VLS Force : Inport  Port=8
  VLP Force : Inport  Port=9
  Convert to Column Vector : MATLAB Function  TreatAsAtomicUnit=on
  Convert to Column Vector1 : MATLAB Function  TreatAsAtomicUnit=on
  Convert to Row Vector : MATLAB Function  TreatAsAtomicUnit=on
  Convert to Row Vector1 : MATLAB Function  TreatAsAtomicUnit=on
  Convert to World Frame : Product  Multiplication=Matrix(*)
  Convert to World Frame 1 : Product  Multiplication=Matrix(*)
  HLP Thruster : Subsystem
  HLS Thruster : Subsystem
  HUP Thruster : Subsystem
  HUS Thruster : Subsystem
  Record : Record  FileSettingsInternal="{\"entries\":[{\"content\":{\"excelSettings\":{\"content\":{},\"type\":\"Streamout.ExcelSettings\"}},\"type\":\"Streamout.FileSettingStorage\",\"uuid\":\"fbe358e9-cb38-49a9-a52b-14c272f6f9b5\"}],\"packageUris\":[\"http://schema.mathworks.com/mf0/streamout_blocks/R2020a\"],\"version\":\"1.0\"}"  SignalsInternal="{\"entries\":[{\"content\":{\"signals\":[{\"content\":{\"blockPath\":[\"Simple_3_Model/Physics Sim/Wrench Calculation/Thruster Forces and Moments/Record\"],\"channel\":[],\"dimensions\":[3,1],\"domain\":\"Simple_3_Model/Physics Sim/Wrench Calculation/Thruster Forces and Moments/Record\",\"hasChildren\":true,\"lineColor\":\"#ff13a6\",\"plots\":[],\"port\":1,\"sid\":[\"\"],\"signalID\":960,\"signalName\":\"Convert to World Frame\"},\"type\":\"RecordBlkView.Signal\",\"uuid\":\"df3d9954-50e1-48b5-9f0b-4bef4188442c\"},{\"content\":{\"blockPath\":[\"Simple_3_Model/Physics Sim/Wrench Calculation/Thruster Forces and Moments/Record\"],\"channel\":[1,1],\"dimensions\":[3,1],\"domain\":\"Simple_3_Model/Physics Sim/Wrench Calculation/Thruster Forces and Moments/Record\",\"lineColor\":\"#a2142f\",\"parentID\":960,\"plots\":[1],\"port\":1,\"sid\":[\"\"],\"signalID\":961,\"signalName\":\"Convert to World Frame\"},\"type\":\"RecordBlkView.Signal\",\"uuid\":\"7ec434f2-e0fb-43f5-a317-6f8c9035a8f6\"},{\"content\":{\"blockPath\":[\"Simple_3_Model/Physics Sim/Wrench Calculation/Thruster Forces and Moments/Record\"],\"channel\":[2,1],\"dimensions\":[3,1],\"domain\":\"Simple_3_Model/Physics Sim/Wrench Calculation/Thruster Forces and Moments/Record\",\"lineColor\":\"#ff13a6\",\"parentID\":960,\"plots\":[1],\"port\":1,\"sid\":[\"\"],\"signalID\":977,\"signalName\":\"Convert to World Frame\"},\"type\":\"RecordBlkView.Signal\",\"uuid\":\"40859199-4621-4e99-a030-950cc582fdb9\"},{\"content\":{\"blockPath\":[\"Simple_3_Model/Physics Sim/Wrench Calculation/Thruster Forces and Moments/Record\"],\"channel\":[3,1],\"dimensions\":[3,1],\"domain\":\"Simple_3_Model/Physics Sim/Wrench Calculation/Thruster Forces and Moments/Record\",\"lineColor\":\"#fe330a\",\"parentID\":960,\"plots\":[1],\"port\":1,\"sid\":[\"\"],\"signalID\":978,\"signalName\":\"Convert to World Frame\"},\"type\":\"RecordBlkView.Signal\",\"uuid\":\"1ba6cf2f-4d61-4c04-b401-df618a56bf72\"}]},\"type\":\"RecordBlkView.InputSignals\",\"uuid\":\"80fbbb56-3033-45a0-b23a-cde89e7f55a2\"}],\"packageUris\":[\"http://schema.mathworks.com/mf0/streamout_blocks/R2020a\"],\"version\":\"1.0\"}"  VisualizationBindings="{\"sparklinesplugin\":{\"info\":[{\"bindingParametersList\":[],\"subplotID\":1}]}}"
  Sum Forces : Sum  Inputs=|++++++++  InputSameDT=on
  Sum Moments : Sum  Inputs=|++++++++
  To World Frame : MATLAB Function  TreatAsAtomicUnit=on
  VLP Thruster : Subsystem
  VLS Thruster : Subsystem
  VUP Thruster : Subsystem
  VUS Thruster : Subsystem
  Forces : Outport
  Moments : Outport  Port=2
  wires:
  HLS Thruster/2(Force) -> Sum Forces/5
  VUS Thruster/1(Moment) -> Sum Moments/1
  VUS Force/1 -> VUS Thruster/1(Thrust Magnitude)
  HLS Thruster/1(Moment) -> Sum Moments/5
  HUS Thruster/1(Moment) -> Sum Moments/3
  HLS Force/1 -> HLS Thruster/1(Thrust Magnitude)
  HUP Thruster/2(Force) -> Sum Forces/4
  VUP Thruster/1(Moment) -> Sum Moments/2
  HLP Thruster/2(Force) -> Sum Forces/6
  HUP Thruster/1(Moment) -> Sum Moments/4
  VLS Force/1 -> VLS Thruster/1(Thrust Magnitude)
  VLP Force/1 -> VLP Thruster/1(Thrust Magnitude)
  VLP Thruster/1(Moment) -> Sum Moments/8
  VUP Thruster/2(Force) -> Sum Forces/2
  HLP Force/1 -> HLP Thruster/1(Thrust Magnitude)
  HUP Force/1 -> HUP Thruster/1(Thrust Magnitude)
  VLS Thruster/2(Force) -> Sum Forces/7
  HUS Thruster/2(Force) -> Sum Forces/3
  Sum Forces/1 -> Convert to Column Vector/1(row)
  VUS Thruster/2(Force) -> Sum Forces/1
  HUS Force/1 -> HUS Thruster/1(Thrust Magnitude)
  VLS Thruster/1(Moment) -> Sum Moments/7
  VUP Force/1 -> VUP Thruster/1(Thrust Magnitude)
  VLP Thruster/2(Force) -> Sum Forces/8
  HLP Thruster/1(Moment) -> Sum Moments/6
  Angular Positions/1 -> To World Frame/1(angularPosition)
  Convert to Row Vector/1(row) -> Forces/1
  Convert to Column Vector/1(column) -> Convert to World Frame/2
  Convert to World Frame/1 -> Record/1, Convert to Row Vector/1(column)
  To World Frame/1(rotation) -> Convert to World Frame 1/1, Convert to World Frame/1
  Convert to World Frame 1/1 -> Convert to Row Vector1/1(column)
  Convert to Row Vector1/1(row) -> Moments/1
  Convert to Column Vector1/1(column) -> Convert to World Frame 1/2
  Sum Moments/1 -> Convert to Column Vector1/1(row)

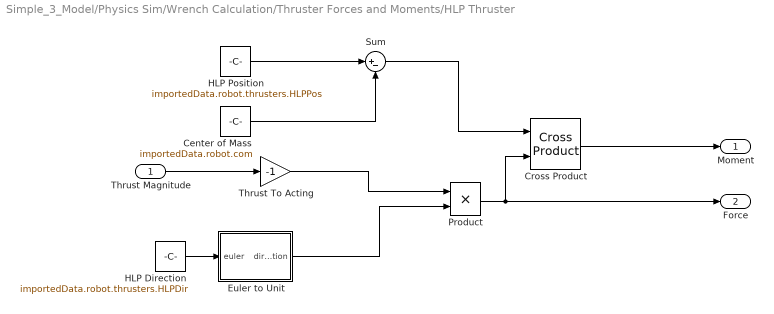
== system Simple_3_Model/Physics Sim/Wrench Calculation/Thruster Forces and Moments/HLP Thruster ==
  Thrust Magnitude : Inport
  Center of Mass : Constant  Value=importedData.robot.com
  Cross Product : matrix_library/Cross Product
  Euler to Unit : MATLAB Function  TreatAsAtomicUnit=on
  HLP Direction : Constant  Value=importedData.robot.thrusters.HLPDir  VectorParams1D=off
  HLP Position : Constant  Value=importedData.robot.thrusters.HLPPos  VectorParams1D=off
  Product : Product
  Sum : Sum  Inputs=|+-
  Thrust To Acting : Gain  Gain=-1
  Moment : Outport
  Force : Outport  Port=2
  wires:
  Product/1 -> Force/1, Cross Product/2
  Cross Product/1 -> Moment/1
  Thrust Magnitude/1 -> Thrust To Acting/1
  HLP Direction/1 -> Euler to Unit/1(euler)
  Euler to Unit/1(direction) -> Product/2
  HLP Position/1 -> Sum/1
  Center of Mass/1 -> Sum/2
  Sum/1 -> Cross Product/1
  Thrust To Acting/1 -> Product/1

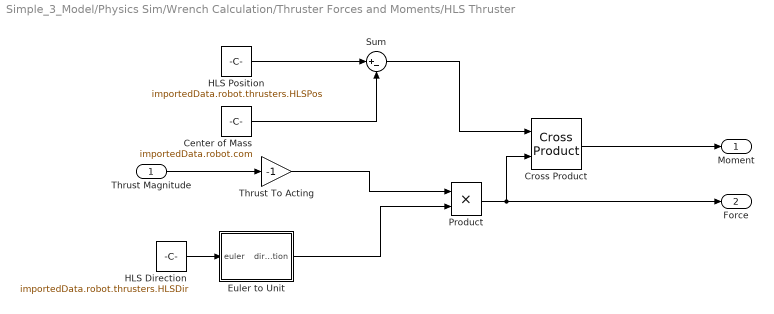
== system Simple_3_Model/Physics Sim/Wrench Calculation/Thruster Forces and Moments/HLS Thruster ==
  Thrust Magnitude : Inport
  Center of Mass : Constant  Value=importedData.robot.com
  Cross Product : matrix_library/Cross Product
  Euler to Unit : MATLAB Function  TreatAsAtomicUnit=on
  HLS Direction : Constant  Value=importedData.robot.thrusters.HLSDir  VectorParams1D=off
  HLS Position : Constant  Value=importedData.robot.thrusters.HLSPos  VectorParams1D=off
  Product : Product
  Sum : Sum  Inputs=|+-
  Thrust To Acting : Gain  Gain=-1
  Moment : Outport
  Force : Outport  Port=2
  wires:
  Product/1 -> Force/1, Cross Product/2
  Cross Product/1 -> Moment/1
  Thrust Magnitude/1 -> Thrust To Acting/1
  HLS Direction/1 -> Euler to Unit/1(euler)
  Euler to Unit/1(direction) -> Product/2
  HLS Position/1 -> Sum/1
  Center of Mass/1 -> Sum/2
  Sum/1 -> Cross Product/1
  Thrust To Acting/1 -> Product/1

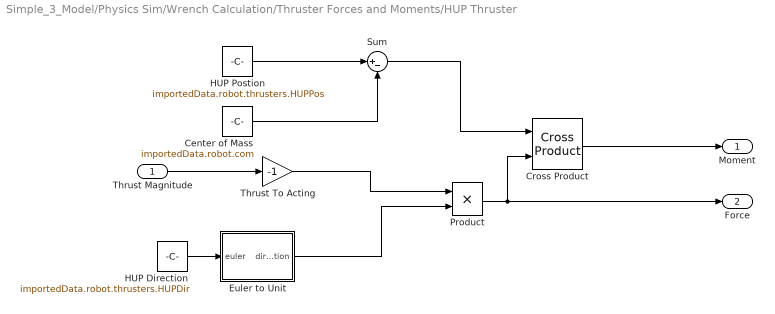
== system Simple_3_Model/Physics Sim/Wrench Calculation/Thruster Forces and Moments/HUP Thruster ==
  Thrust Magnitude : Inport
  Center of Mass : Constant  Value=importedData.robot.com
  Cross Product : matrix_library/Cross Product
  Euler to Unit : MATLAB Function  TreatAsAtomicUnit=on
  HUP Direction : Constant  Value=importedData.robot.thrusters.HUPDir  VectorParams1D=off
  HUP Postion : Constant  Value=importedData.robot.thrusters.HUPPos  VectorParams1D=off
  Product : Product
  Sum : Sum  Inputs=|+-
  Thrust To Acting : Gain  Gain=-1
  Moment : Outport
  Force : Outport  Port=2
  wires:
  Product/1 -> Force/1, Cross Product/2
  Cross Product/1 -> Moment/1
  Thrust Magnitude/1 -> Thrust To Acting/1
  HUP Direction/1 -> Euler to Unit/1(euler)
  Euler to Unit/1(direction) -> Product/2
  HUP Postion/1 -> Sum/1
  Center of Mass/1 -> Sum/2
  Sum/1 -> Cross Product/1
  Thrust To Acting/1 -> Product/1

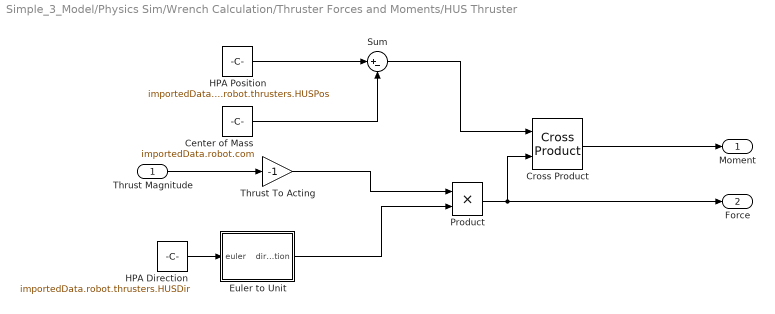
== system Simple_3_Model/Physics Sim/Wrench Calculation/Thruster Forces and Moments/HUS Thruster ==
  Thrust Magnitude : Inport
  Center of Mass : Constant  Value=importedData.robot.com
  Cross Product : matrix_library/Cross Product
  Euler to Unit : MATLAB Function  TreatAsAtomicUnit=on
  HPA Direction : Constant  Value=importedData.robot.thrusters.HUSDir  VectorParams1D=off
  HPA Position : Constant  Value=importedData.robot.thrusters.HUSPos  VectorParams1D=off
  Product : Product
  Sum : Sum  Inputs=|+-
  Thrust To Acting : Gain  Gain=-1
  Moment : Outport
  Force : Outport  Port=2
  wires:
  Product/1 -> Force/1, Cross Product/2
  Cross Product/1 -> Moment/1
  Thrust Magnitude/1 -> Thrust To Acting/1
  HPA Direction/1 -> Euler to Unit/1(euler)
  Euler to Unit/1(direction) -> Product/2
  HPA Position/1 -> Sum/1
  Center of Mass/1 -> Sum/2
  Sum/1 -> Cross Product/1
  Thrust To Acting/1 -> Product/1

== system Simple_3_Model/Physics Sim/Wrench Calculation/Thruster Forces and Moments/VLP Thruster ==
  Thrust Magnitude : Inport
  Center of Mass : Constant  Value=importedData.robot.com
  Cross Product : matrix_library/Cross Product
  Euler to Unit : MATLAB Function  TreatAsAtomicUnit=on
  Product : Product
  Sum : Sum  Inputs=|+-
  Thrust To Acting : Gain  Gain=-1
  VLP Direction : Constant  Value=importedData.robot.thrusters.VLPDir  VectorParams1D=off
  VLP Position : Constant  Value=importedData.robot.thrusters.VLPPos  VectorParams1D=off
  Moment : Outport
  Force : Outport  Port=2
  wires:
  Product/1 -> Force/1, Cross Product/2
  Cross Product/1 -> Moment/1
  Thrust Magnitude/1 -> Thrust To Acting/1
  VLP Direction/1 -> Euler to Unit/1(euler)
  Euler to Unit/1(direction) -> Product/2
  VLP Position/1 -> Sum/1
  Center of Mass/1 -> Sum/2
  Sum/1 -> Cross Product/1
  Thrust To Acting/1 -> Product/1

== system Simple_3_Model/Physics Sim/Wrench Calculation/Thruster Forces and Moments/VLS Thruster ==
  Thrust Magnitude : Inport
  Center of Mass : Constant  Value=importedData.robot.com
  Cross Product : matrix_library/Cross Product
  Euler to Unit : MATLAB Function  TreatAsAtomicUnit=on
  Product : Product
  Sum : Sum  Inputs=|+-
  Thrust To Acting : Gain  Gain=-1
  VLS Direction : Constant  Value=importedData.robot.thrusters.VLSDir  VectorParams1D=off
  VLS Position : Constant  Value=importedData.robot.thrusters.VLSPos  VectorParams1D=off
  Moment : Outport
  Force : Outport  Port=2
  wires:
  Product/1 -> Force/1, Cross Product/2
  Cross Product/1 -> Moment/1
  Thrust Magnitude/1 -> Thrust To Acting/1
  VLS Direction/1 -> Euler to Unit/1(euler)
  Euler to Unit/1(direction) -> Product/2
  VLS Position/1 -> Sum/1
  Center of Mass/1 -> Sum/2
  Sum/1 -> Cross Product/1
  Thrust To Acting/1 -> Product/1

== system Simple_3_Model/Physics Sim/Wrench Calculation/Thruster Forces and Moments/VUP Thruster ==
  Thrust Magnitude : Inport
  Center of Mass : Constant  Value=importedData.robot.com
  Cross Product : matrix_library/Cross Product
  Euler to Unit : MATLAB Function  TreatAsAtomicUnit=on
  HSA Direction : Constant  Value=importedData.robot.thrusters.VUPDir  VectorParams1D=off
  HSA Position : Constant  Value=importedData.robot.thrusters.VUPPos  VectorParams1D=off
  Product : Product
  Sum : Sum  Inputs=|+-
  Thrust To Acting : Gain  Gain=-1
  Moment : Outport
  Force : Outport  Port=2
  wires:
  Product/1 -> Force/1, Cross Product/2
  Cross Product/1 -> Moment/1
  Thrust Magnitude/1 -> Thrust To Acting/1
  HSA Direction/1 -> Euler to Unit/1(euler)
  Euler to Unit/1(direction) -> Product/2
  HSA Position/1 -> Sum/1
  Center of Mass/1 -> Sum/2
  Sum/1 -> Cross Product/1
  Thrust To Acting/1 -> Product/1

== system Simple_3_Model/Physics Sim/Wrench Calculation/Thruster Forces and Moments/VUS Thruster ==
  Thrust Magnitude : Inport
  Center of Mass : Constant  Value=importedData.robot.com
  Cross Product : matrix_library/Cross Product
  Euler to Unit : MATLAB Function  TreatAsAtomicUnit=on
  Product : Product
  Sum : Sum  Inputs=|+-
  Thrust To Acting : Gain  Gain=-1
  VUS Direction : Constant  Value=importedData.robot.thrusters.VUSDir  VectorParams1D=off
  VUS Position : Constant  Value=importedData.robot.thrusters.VUSPos  VectorParams1D=off
  Moment : Outport
  Force : Outport  Port=2
  wires:
  Product/1 -> Force/1, Cross Product/2
  Cross Product/1 -> Moment/1
  Thrust Magnitude/1 -> Thrust To Acting/1
  VUS Direction/1 -> Euler to Unit/1(euler)
  Euler to Unit/1(direction) -> Product/2
  VUS Position/1 -> Sum/1
  Center of Mass/1 -> Sum/2
  Sum/1 -> Cross Product/1
  Thrust To Acting/1 -> Product/1

== matlab function Simple_3_Model/Physics Sim/Wrench Calculation/Linear Drag/Row to Column Vector ==
  data: row input; column output
function column = fcn(row)

column = [row(1); row(2); row(3)];

== matlab function Simple_3_Model/Physics Sim/Wrench Calculation/Thruster Forces and Moments/VUP Thruster/Euler to Unit ==
  data: euler input; direction output
function direction = fcn(euler)

directionCol = eul2rotm(euler, "XYZ") * [1; 0; 0];
direction = [directionCol(1,1), directionCol(2,1), directionCol(3,1)];

== matlab function Simple_3_Model/Physics Sim/Wrench Calculation/Thruster Forces and Moments/HUS Thruster/Euler to Unit ==
  data: euler input; direction output
function direction = fcn(euler)

directionCol = eul2rotm(euler, "XYZ") * [1; 0; 0];
direction = [directionCol(1,1), directionCol(2,1), directionCol(3,1)];

== matlab function Simple_3_Model/Physics Sim/Wrench Calculation/Thruster Forces and Moments/HUP Thruster/Euler to Unit ==
  data: euler input; direction output
function direction = fcn(euler)

directionCol = eul2rotm(euler, "XYZ") * [1; 0; 0];
direction = [directionCol(1,1), directionCol(2,1), directionCol(3,1)];

== matlab function Simple_3_Model/Physics Sim/Wrench Calculation/Thruster Forces and Moments/HLS Thruster/Euler to Unit ==
  data: euler input; direction output
function direction = fcn(euler)

directionCol = eul2rotm(euler, "XYZ") * [1; 0; 0];
direction = [directionCol(1,1), directionCol(2,1), directionCol(3,1)];

== matlab function Simple_3_Model/Physics Sim/Wrench Calculation/Thruster Forces and Moments/HLP Thruster/Euler to Unit ==
  data: euler input; direction output
function direction = fcn(euler)

directionCol = eul2rotm(euler, "XYZ") * [1; 0; 0];
direction = [directionCol(1,1), directionCol(2,1), directionCol(3,1)];

== matlab function Simple_3_Model/Physics Sim/Wrench Calculation/Thruster Forces and Moments/VLS Thruster/Euler to Unit ==
  data: euler input; direction output
function direction = fcn(euler)

directionCol = eul2rotm(euler, "XYZ") * [1; 0; 0];
direction = [directionCol(1,1), directionCol(2,1), directionCol(3,1)];

== matlab function Simple_3_Model/Physics Sim/Wrench Calculation/Thruster Forces and Moments/VLP Thruster/Euler to Unit ==
  data: euler input; direction output
function direction = fcn(euler)

directionCol = eul2rotm(euler, "XYZ") * [1; 0; 0];
direction = [directionCol(1,1), directionCol(2,1), directionCol(3,1)];

== matlab function Simple_3_Model/Physics Sim/Wrench Calculation/Gravity/Create Vector ==
  data: magnitude input; vector output
function vector = fcn(magnitude)

vector = [0, 0, magnitude];

== matlab function Simple_3_Model/Physics Sim/Wrench Calculation/Thruster Forces and Moments/To World Frame ==
  data: angularPosition input; rotation output
function rotation  = fcn(angularPosition)

rotationToRobot = eul2rotm([deg2rad(angularPosition(1)), deg2rad(angularPosition(2)), deg2rad(angularPosition(3))]); %create the rotation matrix to robot frame

rotation = transpose(rotationToRobot);

== matlab function Simple_3_Model/Physics Sim/Wrench Calculation/Thruster Forces and Moments/Convert to Column Vector ==
  data: row input; column output
function column = fcn(row)

column = [row(1); row(2); row(3)];

== matlab function Simple_3_Model/Physics Sim/Wrench Calculation/Linear Drag/Create Rotation Matrix ==
  data: inverse output; angularPosition input; rotation output
function [inverse, rotation] = fcn(angularPosition)

rotation = eul2rotm([deg2rad(angularPosition(1)), deg2rad(angularPosition(2)), deg2rad(angularPosition(3))]);
inverse = transpose(rotation);

== matlab function Simple_3_Model/Physics Sim/Wrench Calculation/Thruster Forces and Moments/Convert to Row Vector ==
  data: column input; row output
function row = fcn(column)

row = [column(1,1), column(2,1), column(3,1)];

== matlab function Simple_3_Model/Physics Sim/Wrench Calculation/Thruster Forces and Moments/Convert to Column Vector1 ==
  data: row input; column output
function column = fcn(row)

column = [row(1); row(2); row(3)];

== matlab function Simple_3_Model/Physics Sim/Wrench Calculation/Thruster Forces and Moments/Convert to Row Vector1 ==
  data: column input; row output
function row = fcn(column)

row = [column(1,1), column(2,1), column(3,1)];

== matlab function Simple_3_Model/Physics Sim/Wrench Calculation/Gradient Bouyancy/Create Bouancy Vector ==
  data: magnitude input; bouyantForce output
function bouyantForce = fcn(magnitude)

bouyantForce = [0, 0, magnitude];

== matlab function Simple_3_Model/Physics Sim/Wrench Calculation/Linear Drag/Seperate to Components ==
  data: x output; robotFrameVelocity input; y output; z output
function [x, y, z] = fcn(robotFrameVelocity)

x = robotFrameVelocity(1, 1);
y = robotFrameVelocity(2, 1);
z = robotFrameVelocity(3, 1);

== matlab function Simple_3_Model/Physics Sim/Wrench Calculation/Linear Drag/Concatenate Drag ==
  data: x input; velocityVector output; y input; z input
function velocityVector = fcn(x,y,z)

velocityVector = [x; y; z];
